simulink model "sample151"  (Simulink 6.3)
settings: Solver=ode45  StartTime=0.0  StopTime=10.0  RelTol=1e-3
libraries: commdigbbndcpm2 x1, commdigbbndfm2 x1
settings Model: LastModifiedBy=Administrator

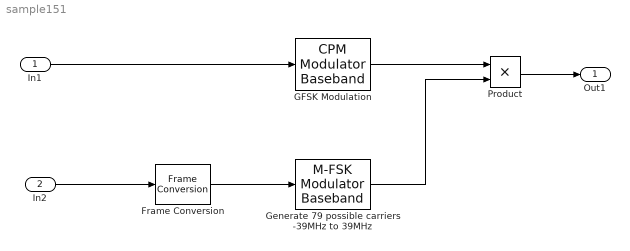
== system sample151 ==
  In1 : Inport
  In2 : Inport  Port=2
  Frame Conversion : FrameConversion
  GFSK Modulation : commdigbbndcpm2/CPM Modulator Baseband  Mnum=4  inputType=Integer  mappingType=Binary  modIdx=0.5  pulseShape=Rectangular  BT=0.3  mainLobePulseLength=1  rollOff=0.2  pulseLength=1  preHistory=1  phaseOffset=0  samplesPerSymbol=8  outDataType=double
  Generate 79 possible carriers -39MHz to 39MHz : commdigbbndfm2/M-FSK Modulator Baseband  M=8  InType=Integer  Enc=Binary  freqSep=6  phaseType=Continuous  numSamp=17  outDataType=double
  Product : Product  RndMeth=Zero
  Out1 : Outport
  wires:
  Product/1 -> Out1/1
  Generate 79 possible carriers -39MHz to 39MHz/1 -> Product/2
  GFSK Modulation/1 -> Product/1
  In1/1 -> GFSK Modulation/1
  Frame Conversion/1 -> Generate 79 possible carriers -39MHz to 39MHz/1
  In2/1 -> Frame Conversion/1
